simulink model "lib"  (Simulink 8.3)
settings: Solver=ode45  StartTime=0.0  StopTime=43  RelTol=1e-3
settings Model: Creator=Administrator  LastModifiedBy=Administrator
settings OptimizationCC: ExpressionDepthLimit=2147483647
settings DebuggingCC: FcnCallInpInsideContextMsg=EnableAllAsWarning

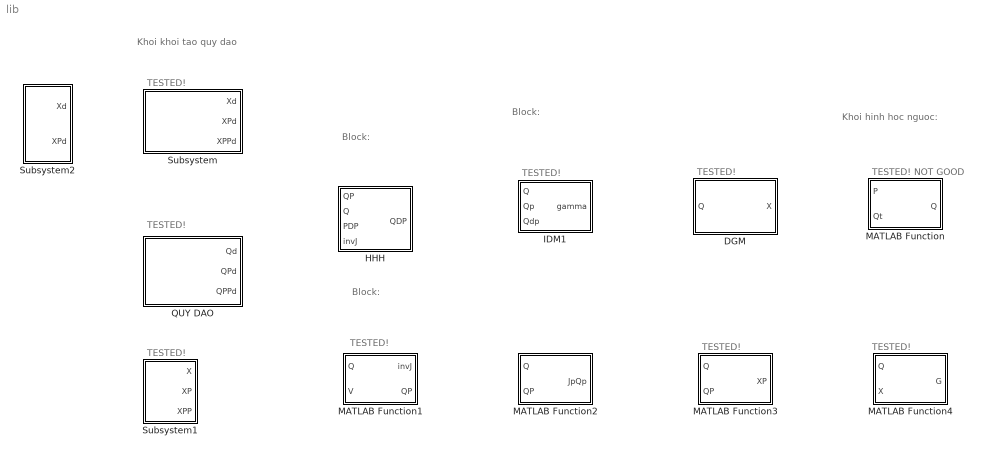
== system lib ==
  note: TESTED!
  note: Khoi khoi tao quy dao
  note: Block:
  note: Khoi hinh hoc nguoc:
  note: Block:
  note: Block:
  note: TESTED!
  note: TESTED!
  note: TESTED!
  note: TESTED! NOT GOOD
  note: TESTED!
  note: TESTED!
  note: TESTED!
  note: TESTED!
  DGM : MATLAB Function  TreatAsAtomicUnit=on
  HHH : MATLAB Function  TreatAsAtomicUnit=on
  IDM1 : MATLAB Function  TreatAsAtomicUnit=on
  MATLAB Function : MATLAB Function  TreatAsAtomicUnit=on
  MATLAB Function1 : MATLAB Function  TreatAsAtomicUnit=on
  MATLAB Function2 : MATLAB Function  TreatAsAtomicUnit=on
  MATLAB Function3 : MATLAB Function  TreatAsAtomicUnit=on
  MATLAB Function4 : MATLAB Function  TreatAsAtomicUnit=on
  QUY DAO : Subsystem
  Subsystem : Subsystem
  Subsystem1 : Subsystem
  Subsystem2 : Subsystem

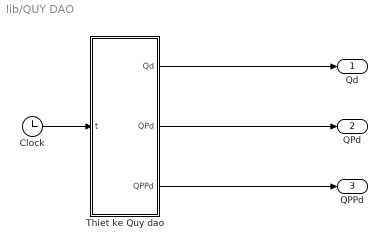
== system lib/QUY DAO ==
  Clock : Clock
  Thiet ke Quy dao : MATLAB Function  TreatAsAtomicUnit=on
  Qd : Outport
  QPd : Outport  Port=2
  QPPd : Outport  Port=3
  wires:
  Thiet ke Quy dao/3(QPPd) -> QPPd/1
  Thiet ke Quy dao/1(Qd) -> Qd/1
  Thiet ke Quy dao/2(QPd) -> QPd/1
  Clock/1 -> Thiet ke Quy dao/1(t)

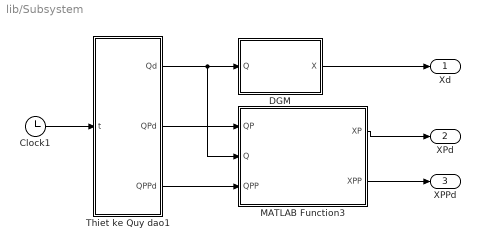
== system lib/Subsystem ==
  Clock1 : Clock
  DGM : MATLAB Function  TreatAsAtomicUnit=on
  MATLAB Function3 : MATLAB Function  TreatAsAtomicUnit=on
  Thiet ke Quy dao1 : MATLAB Function  TreatAsAtomicUnit=on
  Xd : Outport
  XPd : Outport  Port=2
  XPPd : Outport  Port=3
  wires:
  Clock1/1 -> Thiet ke Quy dao1/1(t)
  Thiet ke Quy dao1/1(Qd) -> MATLAB Function3/2(Q), DGM/1(Q)
  DGM/1(X) -> Xd/1
  MATLAB Function3/1(XP) -> XPd/1
  MATLAB Function3/2(XPP) -> XPPd/1
  Thiet ke Quy dao1/3(QPPd) -> MATLAB Function3/3(QPP)
  Thiet ke Quy dao1/2(QPd) -> MATLAB Function3/1(QP)

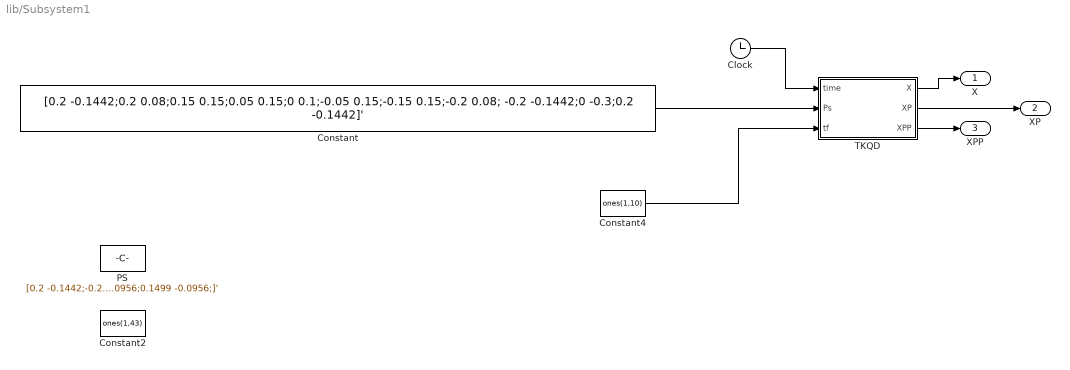
== system lib/Subsystem1 ==
  Clock : Clock
  Constant : Constant  Value=[0.2 -0.1442;0.2 0.08;0.15 0.15;0.05 0.15;0 0.1;-0.05 0.15;-0.15 0.15;-0.2 0.08; -0.2 -0.1442;0 -0.3;0.2 -0.1442]'
  Constant2 : Constant  Value=ones(1,43)
  Constant4 : Constant  Value=ones(1,10)
  PS : Constant  Value=[0.2 -0.1442;-0.2847 -0.0956;-0.2879 0.0916;-0.2673 0.0916;-0.2641 -0.0755;-0.1927 -0.0735;-0.1927 -0.0956;-0.2863 -0.0956;-0.1832 -0.0976;-0.1277 0.0936;-0.1087 0.0916;-0.0436 -0.0956;-0.0627 -0.0956;-0.0849 -0.0352;-0.1451 -0.0372;-0.1594 -0.0936;-0.1816 -0.0936;-0.0262 -0.0996;-0.0262 0.0936; 0.0040 0.0936; 0.0452 -0.0654; 0.0880 0.0916; 0.1134 0.0916; 0.1134 -0.0976; 0.0975 -0.0976; 0.0991 0.0574; 0.0531 -0.0956;0.0341 -0.0956;-0.0071 0.0614;-0.0087 -0.0956;-0.0262 -0.0956; 0.1499 -0.0956; 0.1499 0.0936; 0.2593 0.0936; 0.2578 0.0735; 0.1689 0.0735; 0.1689 0.0131; 0.2530 0.0131; 0.2530 -0.0070; 0.1705 -0.0070; 0.1721 -0.0775; 0.2625 -0.0775; 0.2625 -0.0956;0.1499 -0.0956;]'
  TKQD : MATLAB Function  TreatAsAtomicUnit=on
  X : Outport
  XP : Outport  Port=2
  XPP : Outport  Port=3
  wires:
  TKQD/2(XP) -> XP/1
  TKQD/3(XPP) -> XPP/1
  Clock/1 -> TKQD/1(time)
  TKQD/1(X) -> X/1
  Constant/1 -> TKQD/2(Ps)
  Constant4/1 -> TKQD/3(tf)

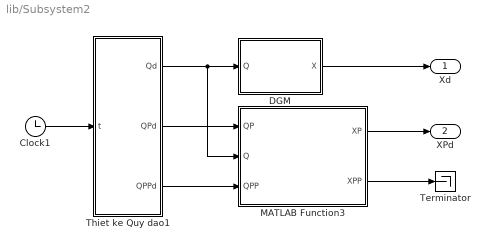
== system lib/Subsystem2 ==
  Clock1 : Clock
  DGM : MATLAB Function  TreatAsAtomicUnit=on
  MATLAB Function3 : MATLAB Function  TreatAsAtomicUnit=on
  Terminator : Terminator
  Thiet ke Quy dao1 : MATLAB Function  TreatAsAtomicUnit=on
  Xd : Outport
  XPd : Outport  Port=2
  wires:
  Clock1/1 -> Thiet ke Quy dao1/1(t)
  Thiet ke Quy dao1/1(Qd) -> MATLAB Function3/2(Q), DGM/1(Q)
  DGM/1(X) -> Xd/1
  MATLAB Function3/1(XP) -> XPd/1
  Thiet ke Quy dao1/3(QPPd) -> MATLAB Function3/3(QPP)
  Thiet ke Quy dao1/2(QPd) -> MATLAB Function3/1(QP)
  MATLAB Function3/2(XPP) -> Terminator/1

== matlab function Subsystem1/TKQD ==
  data: time input double; X output double; Ps input double; tf input double; XP output double; XPP output double
function [X,XP,XPP] = Quintic(time,Ps,tf)
% Calculate trajectory using Quintic polynomial
% r=10*(t/tf)^3-15*(t/tf)^4+6*(t/tf)^5;
% time is clock input
% Ps is the list of point = [P1 P2...]
% tf is the finish time for each interval
n=length(tf);
[k,tk_1] = find(time,tf,n);
if(k==1)
    t=min(time/tf(1),1);
else
    t = min((time-tk_1)/tf(k),1);
end
r=10*t^3-15*t^4+6*t^5;
rd=30*t^2-60*t^3+30*t^4;
r2d=60*t-180*t^2+120*t^3;
D=Ps(:,k+1)-Ps(:,k);
X=Ps(:,k)+r*D;
XP=rd*D;
XPP=r2d*D;
function [k,tk_1]=find(time,tf,n)
t=0;
k=n;
for i=1:n
    tk=t+tf(i);
    if(t<=time)&&(time<tk)
        k=i;
        break;
    end
    t=tk;
    if(i==n)
        t=tk-tf(n);
    end
end
tk_1=t;

== matlab function HHH ==
  data: QP input double; QDP output double; Q input double; PDP input double; invJ input double
function QDP  = HHH(QP,Q,PDP,invJ)
L1=0.2;
L2=0.1442;
q1=Q(1);
q2=Q(2);
c1=cos(q1);
s1=sin(q1);
c12=cos(q1+q2);
s12=sin(q1+q2);
Jp=[-L2*c12*(QP(1)+QP(2))-L1*c1*QP(1), -L2*c12*(QP(1)+QP(2))
    -L2*s12*(QP(1)+QP(2))-L1*s1*QP(1), -L2*s12*(QP(1)+QP(2))];
QDP=invJ*(PDP-Jp*QP);

== matlab function Subsystem2/DGM ==
  data: Q input double; X output double
function X   = f(Q)
%#codegen
% Tested OK
L1 = 0.2;
L2 = 0.1442;
X1 = L1*cos(Q(1)) + L2*cos(Q(1)+Q(2));
X2 = L1*sin(Q(1)) + L2*sin(Q(1)+Q(2));
X = [X1;X2];
end

== matlab function IDM1 ==
  data: Q input double; gamma output double; Qp input double; Qdp input double
function gamma = IDM(Q,Qp,Qdp)
gamma=zeros(2,1);
Q2=Q(2);
Qp1=Qp(1);
Qp2=Qp(2);
Qdp1=Qdp(1);
Qdp2=Qdp(2);
M1 = 1.4899;
L1=0.2;M2=0.464;ZZ1=0.0045;ZZ2=0.00156;
MY2=0;MX2=0.025686;
gamma(1) = Qdp1*(ZZ1 + ZZ2 + L1^2*M2 + 2*L1*MX2*cos(Q2) - 2*L1*MY2*sin(Q2)) + Qdp2*(ZZ2 + L1*MX2*cos(Q2) - L1*MY2*sin(Q2)) - L1*Qp2*(Qp1 + Qp2)*(MY2*cos(Q2) + MX2*sin(Q2)) - L1*Qp1*Qp2*(MY2*cos(Q2) + MX2*sin(Q2));
gamma(2) =  Qdp2*ZZ2 + Qdp1*(ZZ2 + L1*MX2*cos(Q2) - L1*MY2*sin(Q2)) + (L1*Qp1*(MY2*cos(Q2) + MX2*sin(Q2))*(Qp1 - Qp2))/2;
end

== matlab function MATLAB Function ==
  data: P input double; Q output double; Qt input double
function Q = IGM(P,Qt)
L1=0.2;
L2=0.1442;
x=P(1);
y=P(2);
q2=-acos((x^2+y^2-L1^2-L2^2)/2/L1/L2);
q1=cmp(x,y,L1,L2,q2);
k=1;
while ((q1<0)&&(Qt(1)>(2*k-1)*pi/2))
    q1=q1+2*k*pi;
    k=k+1;
end
k=1;
while ((q1>=0)&&(Qt(1)>(2*k+1)*pi/2)&&(q1<=pi))
    q1=q1+2*k*pi;
    k=k+1;
end
Q=[q1;q2];
function q1=cmp(x,y,L1,L2,q2)
L1x=L1+L2*cos(q2);
L1y=L2*sin(q2);
q=[L1x -L1y;L1y L1x]\[x;y];
q1=atan2(q(2),q(1));

== matlab function MATLAB Function1 ==
  data: Q input double; invJ output double; V input double; QP output double
function [invJ,QP] = JT(Q,V)
%#codegen
C1 = cos(Q(1));
S1 = sin(Q(1));
C12 = cos(Q(1)+Q(2));
S12 = sin(Q(1)+Q(2));

L1 = 0.2;
L2 = 0.1442;

J = [-L1*S1-L2*S12, -L2*S12
      L1*C1+L2*C12, L2*C12];
invJ = J^-1;
QP = J^-1*V;

== matlab function MATLAB Function2 ==
  data: Q input double; JpQp output double; QP input double
function JpQp = cmp(Q,QP)
%#codegen
C1 = cos(Q(1));
S1 = sin(Q(1));
C12 = cos(Q(1)+Q(2));
S12 = sin(Q(1)+Q(2));

L1 = 0.2;
L2 = 0.1442;
QP12 = QP(1)+QP(2);
Jp = [-L1*C1*QP(1)-L2*C12*QP12, -L2*C12*QP12
      -L1*S1*QP(1)-L2*S12*QP12, -L2*S12*QP12];
JpQp = Jp*QP;

== matlab function MATLAB Function3 ==
  data: Q input double; XP output double; QP input double
function XP  = JxQP(Q,QP)
%#codegen
% Tested OK
C1 = cos(Q(1));
S1 = sin(Q(1));
C12 = cos(Q(1)+Q(2));
S12 = sin(Q(1)+Q(2));

L1 = 0.2;
L2 = 0.1442;

J1 = [-L1*S1-L2*S12, -L2*S12
      L1*C1+L2*C12, L2*C12];
XP = J1*QP;

== matlab function MATLAB Function4 ==
  data: Q input double; G output double; X input double
function G  = JT(Q,X)
%#codegen
C1 = cos(Q(1));
S1 = sin(Q(1));
C12 = cos(Q(1)+Q(2));
S12 = sin(Q(1)+Q(2));

L1 = 0.2;
L2 = 0.1442;

J = [-L1*S1-L2*S12, -L2*S12
      L1*C1+L2*C12, L2*C12];
G = J.'*X;

== matlab function DGM ==
  data: Q input double; X output double
function X   = f(Q)
%#codegen
% Tested OK
L1 = 0.2;
L2 = 0.1442;
X1 = L1*cos(Q(1)) + L2*cos(Q(1)+Q(2));
X2 = L1*sin(Q(1)) + L2*sin(Q(1)+Q(2));
X = [X1;X2];
end

== matlab function Subsystem/DGM ==
  data: Q input double; X output double
function X   = f(Q)
%#codegen
% Tested OK
L1 = 0.2;
L2 = 0.1442;
X1 = L1*cos(Q(1)) + L2*cos(Q(1)+Q(2));
X2 = L1*sin(Q(1)) + L2*sin(Q(1)+Q(2));
X = [X1;X2];
end

== matlab function Subsystem/MATLAB Function3 ==
  data: QP input double; Q input double; XP output double; QPP input double; XPP output double
function [XP, XPP]  = JxQP(QP,Q,QPP)
%#codegen
C1 = cos(Q(1));
S1 = sin(Q(1));
C12 = cos(Q(1)+Q(2));
S12 = sin(Q(1)+Q(2));

L1 = 0.2;
L2 = 0.1442;

J1 = [-L1*S1-L2*S12, -L2*S12
      L1*C1+L2*C12, L2*C12];
XP = J1*QP;
XPP = J1*QPP;

== matlab function Subsystem/Thiet ke Quy dao1 ==
  data: t input double; Qd output double; QPd output double; QPPd output double
function [Qd, QPd, QPPd] = TKQD(t)
%#codegen
Qd = [sin(t)
      -pi/2*cos(t)];
QPd = [cos(t)
       pi/2*sin(t)];
QPPd = [-sin(t)
       pi/2*cos(t)];

== matlab function QUY DAO/Thiet ke Quy dao ==
  data: t input double; Qd output double; QPd output double; QPPd output double
function [Qd, QPd, QPPd] = TKQD(t)
%#codegen
Qd = [sin(t)
      -pi/2*cos(t)];
QPd = [cos(t)
       pi/2*sin(t)];
QPPd = [-sin(t)
       pi/2*cos(t)];

== matlab function Subsystem2/MATLAB Function3 ==
  data: QP input double; Q input double; XP output double; QPP input double; XPP output double
function [XP, XPP]  = JxQP(QP,Q,QPP)
%#codegen
C1 = cos(Q(1));
S1 = sin(Q(1));
C12 = cos(Q(1)+Q(2));
S12 = sin(Q(1)+Q(2));

L1 = 0.2;
L2 = 0.1442;

J1 = [-L1*S1-L2*S12, -L2*S12
      L1*C1+L2*C12, L2*C12];
XP = J1*QP;
XPP = J1*QPP;

== matlab function Subsystem2/Thiet ke Quy dao1 ==
  data: t input double; Qd output double; QPd output double; QPPd output double
function [Qd, QPd, QPPd] = TKQD(t)
%#codegen
Qd = [sin(t)
      -pi/2*cos(t)];
QPd = [cos(t)
       pi/2*sin(t)];
QPPd = [-sin(t)
       pi/2*cos(t)];
